simulink model "UR06_dynamics_sim"  (R2020b)
settings: Solver=ode45  StartTime=0.0  StopTime=2  RelTol=1e-3
libraries: roblocks x2
settings Model: Creator=stardust  LastModifiedBy=stardust

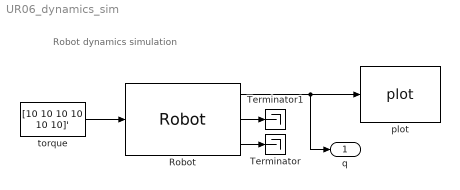
== system UR06_dynamics_sim ==
  note: Robot dynamics simulation
  " torque" : Constant  Value=[10 10 10 10 10 10]'
  Robot : roblocks/Arm/Robot  robot=R  q0=[0 0 0 0 0 0]
  Terminator : Terminator
  Terminator1 : Terminator
  plot : roblocks/Arm/plot  robot=R  fps=25  holdplot=on
  q : Outport
  wires:
  Robot/1 -> plot/1, q/1
  Robot/3 -> Terminator/1
  Robot/2 -> Terminator1/1
  " torque"/1 -> Robot/1
